simulink model "first_order"  (R2016a)
settings: Solver=ode45  StartTime=0.0  StopTime=30  RelTol=1e-3
libraries: simulink x1
settings Model: Creator=86186  LastModifiedBy=86186

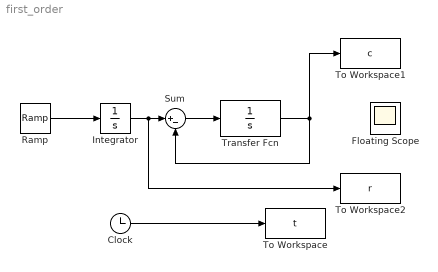
== system first_order ==
  Clock : Clock
  Floating Scope : Scope
      settings: Floating=on
  Integrator : Integrator
  Ramp : simulink/Sources/Ramp  slope=1  start=0  X0=0
  Sum : Sum  Inputs=|+-
  To Workspace : ToWorkspace  VariableName=t  SampleTime=-1
  To Workspace1 : ToWorkspace  VariableName=c  SampleTime=-1
  To Workspace2 : ToWorkspace  VariableName=r  SampleTime=-1
  Transfer Fcn : TransferFcn  Denominator=[1 0]
  wires:
  Sum/1 -> Transfer Fcn/1
  Transfer Fcn/1 -> Sum/2, To Workspace1/1
  Clock/1 -> To Workspace/1
  Ramp/1 -> Integrator/1
  Integrator/1 -> To Workspace2/1, Sum/1
